simulink model "CSTH"  (R2019b)
settings: Solver=ode5  StartTime=0.0  StopTime=700  FixedStep=0.01  RelTol=1e-3
InitFcn:
  | ParamInit
values from neighbouring files (symbols this model uses):
  A = pi*D^2/4    (= 0.0706858347058)    [ParamInit.m]
  Ac = pi*D^2*Hc + pi*D^2/4    (= 0.240331838)    [ParamInit.m]
  Cp = 4190    [ParamInit.m]
  Cpc = 2400    [ParamInit.m]
  g = 9.8    [ParamInit.m]
  H0 = 0.7    [ParamInit.m]
  KL = 125    [ParamInit.m]
  KT = 2.0    (= 2)    [ParamInit.m]
  KvL = 1.5e-5    (= 1.5e-05)    [ParamInit.m]
  KvT = 3e-6    (= 3e-06)    [ParamInit.m]
  KxL = 0.01    [ParamInit.m]
  KxT = 0.01    [ParamInit.m]
  Pcp = 414    [ParamInit.m]
  Pcr = 138    [ParamInit.m]
  Qin = 7e-4    (= 0.0007)    [ParamInit.m]
  Rc = 5.5e7    (= 55000000)    [ParamInit.m]
  rho = 1200    [ParamInit.m]
  rhoC = 800    [ParamInit.m]
  RvT = 50    [ParamInit.m]
  T0 = 38    [ParamInit.m]
  Tci = 900    [ParamInit.m]
  Tin = 24    [ParamInit.m]
  TL = 2    [ParamInit.m]
  TT = 15    [ParamInit.m]
  TvT = 5    [ParamInit.m]
  U = 440    [ParamInit.m]
  UL0 = 71.72    [ParamInit.m]
  UT0 = 89    [ParamInit.m]
  Vc = Hc*pi*((D+2*Wc)^2 - D^2)/4 + Wc*pi*(D + 2*Wc)^2/4    (= 0.0138795563436)    [ParamInit.m]
  XL0 = 0.7172    [ParamInit.m]
  XT0 = 0.89    [ParamInit.m]
  YL0 = 87.48    [ParamInit.m]
  YT0 = 76    [ParamInit.m]
undefined symbols (not defined in the file or in its folder): Tca0
settings Model: Creator=david  LastModifiedBy=david

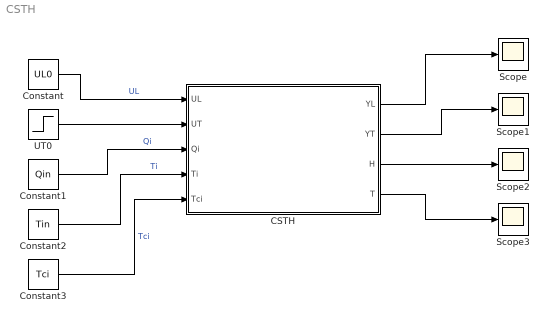
== system CSTH ==
  CSTH : Subsystem
      mask Display: image('$imagefile'); % Use "Edit Image" on toolstrip to change.
  Constant : Constant  Value=UL0
  Constant1 : Constant  Value=Qin
  Constant2 : Constant  Value=Tin
  Constant3 : Constant  Value=Tci
  Scope{,1..3} (4 alike) : Scope
  UT0 : Step  Time=100  Before=UT0  After=UT0+10  SampleTime=0
  wires:
  Constant1/1 -> CSTH/3(Qi)  "Qi"
  Constant2/1 -> CSTH/4(Ti)  "Ti"
  Constant3/1 -> CSTH/5(Tci)  "Tci"
  CSTH/1(YL) -> Scope/1
  CSTH/2(YT) -> Scope1/1
  CSTH/3(H) -> Scope2/1
  CSTH/4(T) -> Scope3/1
  Constant/1 -> CSTH/1(UL)  "UL"
  UT0/1 -> CSTH/2(UT)

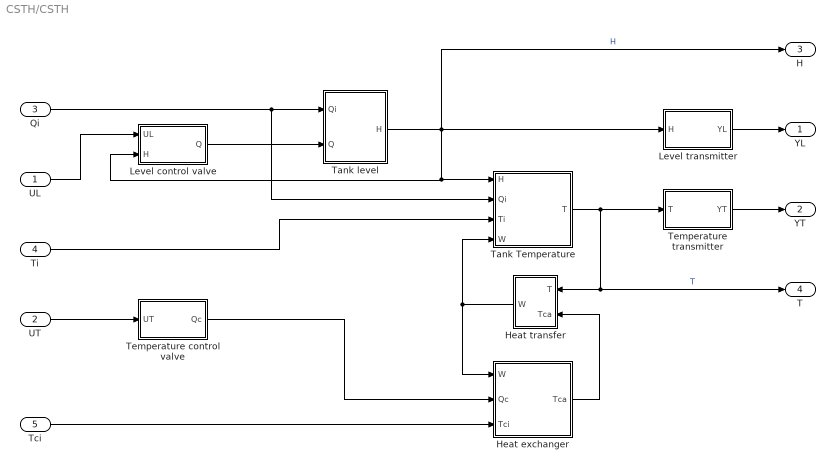
== system CSTH/CSTH ==
  UL : Inport
  UT : Inport  Port=2
  Qi : Inport  Port=3
  Ti : Inport  Port=4
  Tci : Inport  Port=5
  Heat exchanger : Subsystem
  Heat transfer : Subsystem
  Level control valve : Subsystem
  Level transmitter : Subsystem
  Tank Temperature : Subsystem
  Tank level : Subsystem
  Temperature control valve : Subsystem
  Temperature transmitter : Subsystem
  YL : Outport
  YT : Outport  Port=2
  H : Outport  Port=3
  T : Outport  Port=4
  wires:
  Level transmitter/1(YL) -> YL/1
  UT/1 -> Temperature control valve/1(UT)
  Tank level/1(H) -> H/1, Level transmitter/1(H), Tank Temperature/1(H), Level control valve/2(H)  "H"
  Heat exchanger/1(Tca) -> Heat transfer/2(Tca)
  Level control valve/1(Q) -> Tank level/2(Q)
  Heat transfer/1(W) -> Heat exchanger/1(W), Tank Temperature/4(W)
  Temperature control valve/1(Qc) -> Heat exchanger/2(Qc)
  UL/1 -> Level control valve/1(UL)
  Qi/1 -> Tank Temperature/2(Qi), Tank level/1(Qi)
  Tank Temperature/1(T) -> Temperature transmitter/1(T), T/1, Heat transfer/1(T)  "T"
  Temperature transmitter/1(YT) -> YT/1
  Ti/1 -> Tank Temperature/3(Ti)
  Tci/1 -> Heat exchanger/3(Tci)

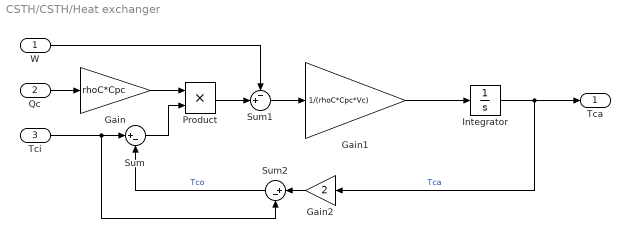
== system CSTH/CSTH/Heat exchanger ==
  W : Inport
  Qc : Inport  Port=2
  Tci : Inport  Port=3
  Gain : Gain  Gain=rhoC*Cpc
  Gain1 : Gain  Gain=1/(rhoC*Cpc*Vc)
  Gain2 : Gain  Gain=2
  Integrator : Integrator  InitialCondition=Tca0  ContinuousStateAttributes='Tca'
  Product : Product
  Sum : Sum  Inputs=|+-
  Sum1 : Sum  Inputs=-+|
  Sum2 : Sum  Inputs=|+-
  Tca : Outport
  wires:
  Tci/1 -> Sum2/2, Sum/1
  Qc/1 -> Gain/1
  Sum/1 -> Product/2
  W/1 -> Sum1/1
  Integrator/1 -> Gain2/1, Tca/1  "Tca"
  Product/1 -> Sum1/2
  Gain/1 -> Product/1
  Sum1/1 -> Gain1/1
  Gain1/1 -> Integrator/1
  Gain2/1 -> Sum2/1
  Sum2/1 -> Sum/2  "Tco"

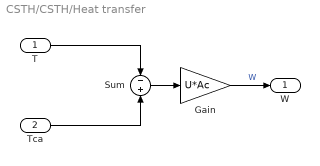
== system CSTH/CSTH/Heat transfer ==
  T : Inport
  Tca : Inport  Port=2
  Gain : Gain  Gain=U*Ac
  Sum : Sum  Inputs=-|+
  W : Outport
  wires:
  T/1 -> Sum/1
  Tca/1 -> Sum/2
  Gain/1 -> W/1  "W"
  Sum/1 -> Gain/1

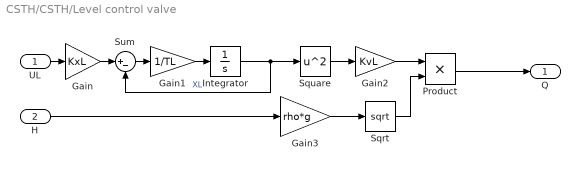
== system CSTH/CSTH/Level control valve ==
  UL : Inport
  H : Inport  Port=2
  Gain : Gain  Gain=KxL
  Gain1 : Gain  Gain=1/TL
  Gain2 : Gain  Gain=KvL
  Gain3 : Gain  Gain=rho*g
  Integrator : Integrator  InitialCondition=XL0
  Product : Product
  Sqrt : Sqrt  SaturateOnIntegerOverflow=on
  Square : Math  Operator=square  SignedPower=off  SaturateOnIntegerOverflow=on
  Sum : Sum  Inputs=|+-
  Q : Outport
  wires:
  Sum/1 -> Gain1/1
  Gain/1 -> Sum/1
  Integrator/1 -> Square/1, Sum/2  "XL"
  UL/1 -> Gain/1
  Gain1/1 -> Integrator/1
  Square/1 -> Gain2/1
  Gain2/1 -> Product/1
  Product/1 -> Q/1
  Sqrt/1 -> Product/2
  H/1 -> Gain3/1
  Gain3/1 -> Sqrt/1

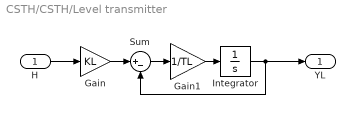
== system CSTH/CSTH/Level transmitter ==
  H : Inport
  Gain : Gain  Gain=KL
  Gain1 : Gain  Gain=1/TL
  Integrator : Integrator  InitialCondition=YL0
  Sum : Sum  Inputs=|+-
  YL : Outport
  wires:
  Sum/1 -> Gain1/1
  Gain/1 -> Sum/1
  Integrator/1 -> YL/1, Sum/2
  H/1 -> Gain/1
  Gain1/1 -> Integrator/1

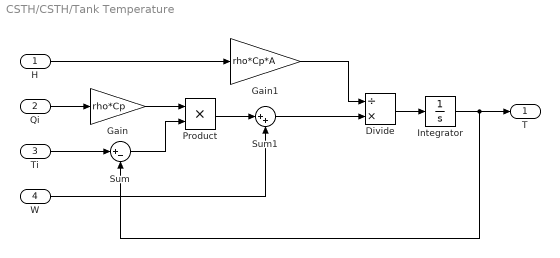
== system CSTH/CSTH/Tank Temperature ==
  H : Inport
  Qi : Inport  Port=2
  Ti : Inport  Port=3
  W : Inport  Port=4
  Divide : Product  Inputs=/*
  Gain : Gain  Gain=rho*Cp
  Gain1 : Gain  Gain=rho*Cp*A
  Integrator : Integrator  InitialCondition=T0
  Product : Product
  Sum : Sum  Inputs=|+-
  Sum1 : Sum  Inputs=|++
  T : Outport
  wires:
  Ti/1 -> Sum/1
  W/1 -> Sum1/2
  Sum/1 -> Product/2
  Product/1 -> Sum1/1
  Qi/1 -> Gain/1
  Gain/1 -> Product/1
  Divide/1 -> Integrator/1
  Integrator/1 -> Sum/2, T/1
  H/1 -> Gain1/1
  Gain1/1 -> Divide/1
  Sum1/1 -> Divide/2

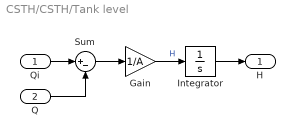
== system CSTH/CSTH/Tank level ==
  Qi : Inport
  Q : Inport  Port=2
  Gain : Gain  Gain=1/A
  Integrator : Integrator  InitialCondition=H0
  Sum : Sum  Inputs=|+-
  H : Outport
  wires:
  Q/1 -> Sum/2
  Qi/1 -> Sum/1
  Sum/1 -> Gain/1
  Gain/1 -> Integrator/1  "H"
  Integrator/1 -> H/1

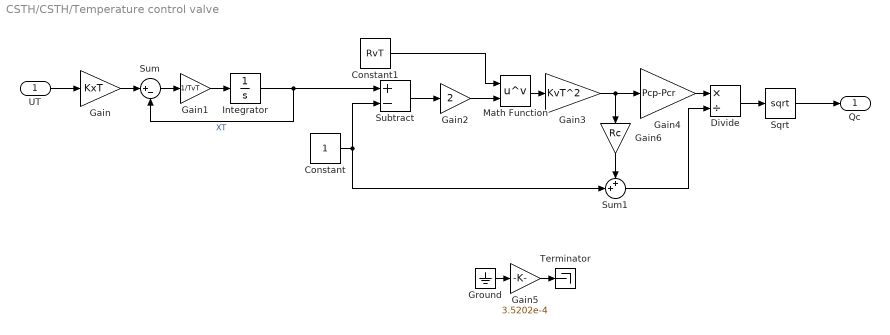
== system CSTH/CSTH/Temperature control valve ==
  UT : Inport
  Constant : Constant
  Constant1 : Constant  Value=RvT
  Divide : Product  Inputs=*/
  Gain : Gain  Gain=KxT
  Gain1 : Gain  Gain=1/TvT
  Gain2 : Gain  Gain=2
  Gain3 : Gain  Gain=KvT^2
  Gain4 : Gain  Gain=Pcp-Pcr
  Gain5 : Gain  Gain=3.5202e-4
  Gain6 : Gain  Gain=Rc
  Ground : Ground
  Integrator : Integrator  InitialCondition=XT0
  Math Function : Math  Operator=pow  SignedPower=off  SaturateOnIntegerOverflow=on
  Sqrt : Sqrt  SaturateOnIntegerOverflow=on
  Subtract : Sum  Inputs=+-
  Sum : Sum  Inputs=|+-
  Sum1 : Sum  Inputs=++|
  Terminator : Terminator
  Qc : Outport
  wires:
  Gain1/1 -> Integrator/1
  UT/1 -> Gain/1
  Integrator/1 -> Sum/2, Subtract/1  "XT"
  Gain/1 -> Sum/1
  Sum/1 -> Gain1/1
  Constant/1 -> Sum1/2, Subtract/2
  Constant1/1 -> Math Function/1
  Subtract/1 -> Gain2/1
  Gain2/1 -> Math Function/2
  Math Function/1 -> Gain3/1
  Gain3/1 -> Gain6/1, Gain4/1
  Gain4/1 -> Divide/1
  Sum1/1 -> Divide/2
  Divide/1 -> Sqrt/1
  Gain6/1 -> Sum1/1
  Sqrt/1 -> Qc/1
  Ground/1 -> Gain5/1
  Gain5/1 -> Terminator/1

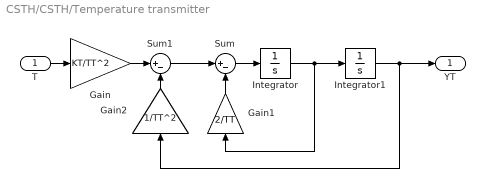
== system CSTH/CSTH/Temperature transmitter ==
  T : Inport
  Gain : Gain  Gain=KT/TT^2
  Gain1 : Gain  Gain=2/TT
  Gain2 : Gain  Gain=1/TT^2
  Integrator : Integrator
  Integrator1 : Integrator  InitialCondition=YT0
  Sum : Sum  Inputs=|+-
  Sum1 : Sum  Inputs=|+-
  YT : Outport
  wires:
  Sum/1 -> Integrator/1
  Gain/1 -> Sum1/1
  Integrator/1 -> Gain1/1, Integrator1/1
  Gain1/1 -> Sum/2
  T/1 -> Gain/1
  Integrator1/1 -> YT/1, Gain2/1
  Sum1/1 -> Sum/1
  Gain2/1 -> Sum1/2
